simulink model "MPC_mobile_base_KIN_IPOPT_poly5"  (R2018b)
settings: Solver=ode4  StartTime=0.0  StopTime=inf  FixedStep=Tsample  RelTol=1e-3
values from neighbouring files (symbols this model uses):
  disturb = 6    [traj_cones.m]
  N = 10    [STEP.m]    (also in WS.mat = 20; solver_NLP.m = evalin('base', 'N'); solver_NLP1.m = evalin('base', 'N'); traiettoria2.m = 20)
  T = 0.2    [STEP.m]    (also in WS.mat = 0.25; traiettoria2.m = 0.25; traiettoria3.m = 0.25; traiettoria4.m)
  Tsample = 0.01    [STEP.m]    (also in WS.mat; traiettoria2.m; traiettoria3.m; traiettoria4.m)
  xd = [linspace(0,5,length(tt));0.5*ones(size(tt));zeros(size(tt))]    [STEP.m]    (also in WS.mat = [0 0 0 0 0 0.000163624617374 0.0189659089948 3.10328963012e-; traiettoria2.m = [x;y+ones(size(y))*0;th]; traiettoria3.m = [x;y+ones(size(y))*0.3;th]; traiettoria4.m = [x;y+ones(size(y))*0;th])
undefined symbols (not defined in the file or in its folder): DiscIntNeverNeededParam
libraries: simulink x2, templibrary x1
settings Model: Creator=francesco  LastModifiedBy=raffaele

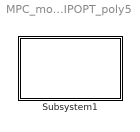
== system MPC_mobile_base_KIN_IPOPT_poly5 ==
  Subsystem1 : Subsystem  InitFcn=init

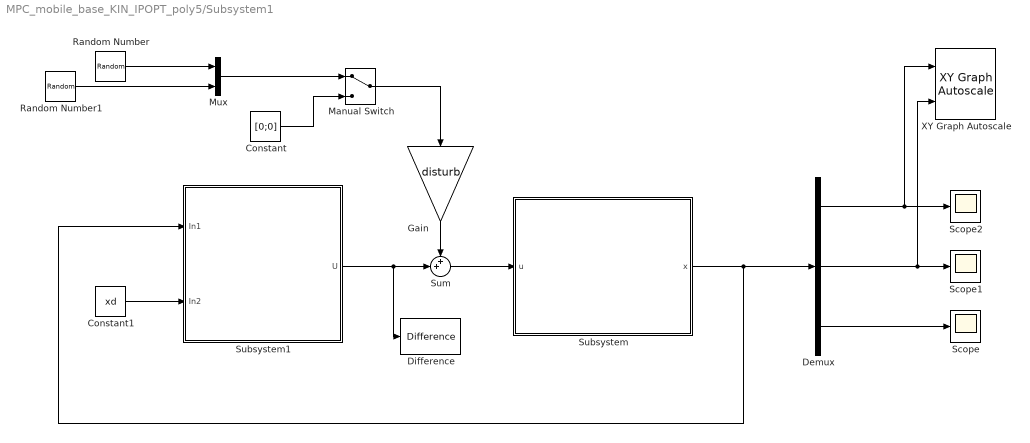
== system MPC_mobile_base_KIN_IPOPT_poly5/Subsystem1 ==
  Constant : Constant  Value=[0;0]
  Constant1 : Constant  Value=xd
  Demux : Demux  Outputs=3
  Difference : simulink/Discrete/Difference  ICPrevInput=0.0  OutMin=[]  OutMax=[]  OutDataType=fixdt(1, 16)  OutScaling=2^-10  DoSatur=off
  Gain : Gain  Gain=disturb
  Manual Switch : ManualSwitch
  Mux : Mux  Inputs=2
  Random Number : RandomNumber  Variance=0.01  SampleTime=T
  Random Number1 : RandomNumber  Variance=0.01  SampleTime=T
  Scope : Scope
  Scope1 : Scope
  Scope2 : Scope
  Subsystem : Subsystem
      mask Display: disp('{\bf\fontsize{10}KINEMATIC SYSTEM}', 'texmode','on');
  Subsystem1 : Subsystem
  Sum : Sum  Inputs=++|
  XY Graph Autoscale : templibrary/XY Graph  Autoscale  xmin=-1  xmax=1  ymin=-1  ymax=1  st=-1
  wires:
  Subsystem/1(x) -> Demux/1, Subsystem1/1(In1)
  Demux/1 -> XY Graph Autoscale/1, Scope2/1
  Demux/3 -> Scope/1
  Demux/2 -> XY Graph Autoscale/2, Scope1/1
  Subsystem1/1(U) -> Sum/2, Difference/1
  Constant1/1 -> Subsystem1/2(In2)
  Sum/1 -> Subsystem/1(u)
  Constant/1 -> Manual Switch/2
  Random Number/1 -> Mux/1
  Random Number1/1 -> Mux/2
  Mux/1 -> Manual Switch/1
  Manual Switch/1 -> Gain/1
  Gain/1 -> Sum/1

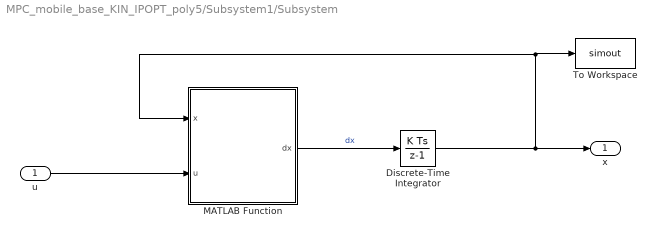
== system MPC_mobile_base_KIN_IPOPT_poly5/Subsystem1/Subsystem ==
  u : Inport
  Discrete-Time Integrator : DiscreteIntegrator  InitialCondition=[-0.15 0.1 0]  SampleTime=Tsample  ICPrevOutput=DiscIntNeverNeededParam  ICPrevScaledInput=DiscIntNeverNeededParam
  MATLAB Function : MATLAB Function  TreatAsAtomicUnit=on
  To Workspace : ToWorkspace  VariableName=simout  SaveFormat=Timeseries  SampleTime=T
  x : Outport  SampleTime=Tsample
  wires:
  u/1 -> MATLAB Function/2(u)
  MATLAB Function/1(dx) -> Discrete-Time Integrator/1  "dx"
  Discrete-Time Integrator/1 -> MATLAB Function/1(x), To Workspace/1, x/1

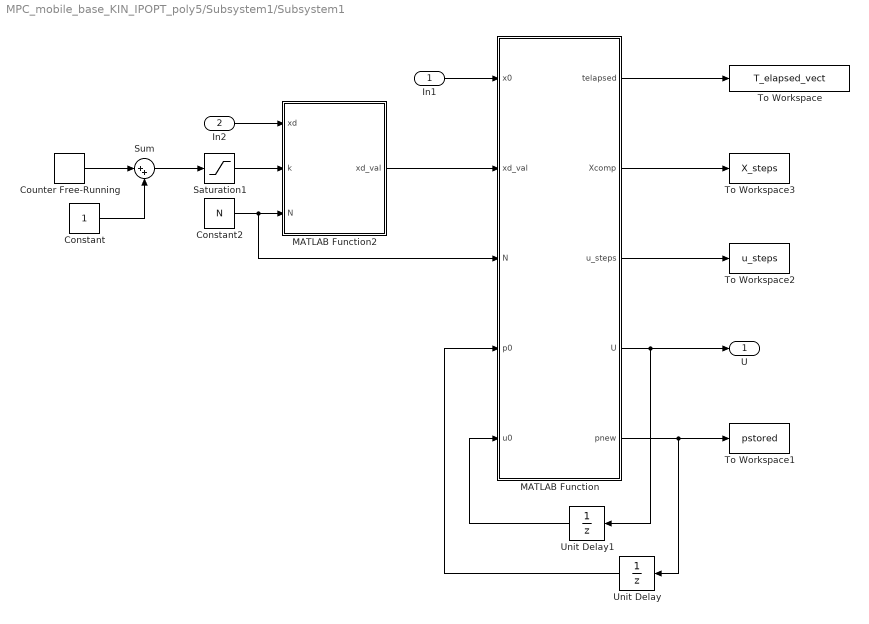
== system MPC_mobile_base_KIN_IPOPT_poly5/Subsystem1/Subsystem1 ==
  In1 : Inport
  In2 : Inport  Port=2
  Constant : Constant
  Constant2 : Constant  Value=N
  Counter Free-Running : simulink/Sources/Counter Free-Running  NumBits=12  tsamp=T
  MATLAB Function : MATLAB Function  TreatAsAtomicUnit=on
  MATLAB Function2 : MATLAB Function  TreatAsAtomicUnit=on
  Saturation1 : Saturate  UpperLimit=size(xd,2)
  Sum : Sum  Inputs=|++
  To Workspace : ToWorkspace  VariableName=T_elapsed_vect  SampleTime=T
  To Workspace1 : ToWorkspace  VariableName=pstored  SampleTime=-1
  To Workspace2 : ToWorkspace  VariableName=u_steps  SaveFormat=Structure  SampleTime=-1
  To Workspace3 : ToWorkspace  VariableName=X_steps  SaveFormat=Structure  SampleTime=-1
  Unit Delay : UnitDelay  InitialCondition=[0 0 0 0 0 0 0 0 0 0 0 0 ].'  SampleTime=T
  Unit Delay1 : UnitDelay  InitialCondition=[0 0].'  SampleTime=T
  U : Outport
  wires:
  Counter Free-Running/1 -> Sum/1
  MATLAB Function/5(pnew) -> To Workspace1/1, Unit Delay/1
  Sum/1 -> Saturation1/1
  Constant/1 -> Sum/2
  In1/1 -> MATLAB Function/1(x0)
  Constant2/1 -> MATLAB Function/3(N), MATLAB Function2/3(N)
  In2/1 -> MATLAB Function2/1(xd)
  MATLAB Function/4(U) -> Unit Delay1/1, U/1
  Unit Delay/1 -> MATLAB Function/4(p0)
  Saturation1/1 -> MATLAB Function2/2(k)
  MATLAB Function2/1(xd_val) -> MATLAB Function/2(xd_val)
  MATLAB Function/1(telapsed) -> To Workspace/1
  Unit Delay1/1 -> MATLAB Function/5(u0)
  MATLAB Function/3(u_steps) -> To Workspace2/1
  MATLAB Function/2(Xcomp) -> To Workspace3/1

== matlab function MPC_mobile_base_KIN_IPOPT_poly5/Subsystem1/Subsystem1/MATLAB Function ==
  settings: updateMethod=DISCRETE  sampleTime=T
  data: telapsed output; Xcomp output size=[3,N+1]; u_steps output size=[3,N]; U output; x0 input; pnew output; xd_val input; N input; p0 input; u0 input
function [telapsed,Xcomp,u_steps,U,pnew] = fnc(x0,xd_val,N,p0,u0)

telapsed=0;
u_steps=zeros(2,N);

coder.extrinsic('solver_NLP1');

pnew=zeros(12,1);
U=zeros(2,1);
Xcomp=zeros(3,N);

[pnew, U, u_steps, Xcomp, telapsed] = solver_NLP1(xd_val,p0,x0,u0);


end

== matlab function MPC_mobile_base_KIN_IPOPT_poly5/Subsystem1/Subsystem1/MATLAB Function2 ==
  settings: updateMethod=DISCRETE  sampleTime=T
  data: xd input; k input; N input; xd_val output size=[3,N]
function xd_val = fcn(xd,k,N)

xd_val=zeros(3,N);

if size(xd,2)-k>N-1
h=xd(:,k+1:k+N);
      
else
h=[xd(:,k+1:end) xd(:,end)*ones(1,N-(size(xd,2)-k))];

end
xd_val = h;

end

== matlab function MPC_mobile_base_KIN_IPOPT_poly5/Subsystem1/Subsystem/MATLAB Function ==
  settings: updateMethod=DISCRETE  sampleTime=Tsample
  data: x input; dx output; u input size=[2 1]
function dx = sys_dynamics(x,u)
dx=zeros(1,3);
dx(1,1)=u(1,1)*cos(x(3));
dx(1,2)=u(1,1)*sin(x(3));
dx(1,3)=u(2,1);

end
